simulink model "power_V__"  (R2019b)
settings: Solver=ode23tb  StartTime=0.0  StopTime=24*60*60  RelTol=1e-4  AbsTol=5e-3
PreLoadFcn:
  | % Load Data and Parameters used by the model:
  | load power_V2G.mat
  | to=0.1;
undefined symbols (not defined in the file): A, B, C, D1, Dd, Delta, j, V2G
libraries: powerlib x37, powerlib_meascontrol x5, simulink x5, spsDieselMotorModel x1, sps_avr x1, V2Glib x1, simulink_extras x1
(part 1 of 2)
settings Model: SimulationMode=accelerator  ExtModeTrigDuration=100  Creator=MathWorks  LastModifiedBy=mdeat
settings SolverCC: AutoScaleAbsTol=off  MaxConsecutiveMinStep=1e6
settings DataIOCC: LimitDataPoints=on  SaveFormat=Array  ReturnWorkspaceOutputs=off
settings OptimizationCC: BlockReduction=off  BooleanDataType=off  EfficientMapNaN2IntZero=off  LifeSpan=inf
settings DebuggingCC: SaveWithParameterizedLinksMsg=none  UnderspecifiedInitializationDetection=Classic  MergeDetectMultiDrivingBlocksExec=none  SignalResolutionControl=TryResolveAllWithWarning  AllowSymbolicDim=off  SFUnexpectedBacktrackingDiag=warning  SFNoUnconditionalDefaultTransitionDiag=warning  SFExecutionAtInitializationDiag=none  ArithmeticOperatorsInVariantConditions=warning
settings HardwareCC: ProdBitPerPointer=32  ProdBitPerSizeT=32  ProdBitPerPtrDiffT=32  ProdLargestAtomicFloat=None  ProdIntDivRoundTo=Undefined  ProdEndianess=Unspecified  ProdWordSize=32  ProdHWDeviceType=32-bit Generic  TargetBitPerPointer=64  TargetBitPerSizeT=64  TargetBitPerPtrDiffT=64  TargetLongLongMode=on  TargetIntDivRoundTo=Zero  TargetEndianess=LittleEndian  TargetWordSize=64  TargetHWDeviceType=MATLAB Host  ProdEqTarget=off
settings ModelReferenceCC: PropagateSignalLabelsOutOfModel=off
settings SFSimCC: SimUseLocalCustomCode=off  CustomCodeUndefinedFunction=UseInterfaceOnly
settings RTWCC: RTWUseLocalCustomCode=off
settings CodeAppCC: MaxIdLength=128
settings GRTTargetCC: TargetLangStandard=C89/C90 (ANSI)  CombineOutputUpdateFcns=off  GRTInterface=on
settings ConfigComp: CovMetricSettings=dw  CovHtmlReporting=on  CovSaveCumulativeToWorkspaceVar=on  CovSaveSingleToWorkspaceVar=on  CovExternalEMLEnable=off  CovSFcnEnable=off
settings SimscapeCC: SimscapeNormalizeSystem=off

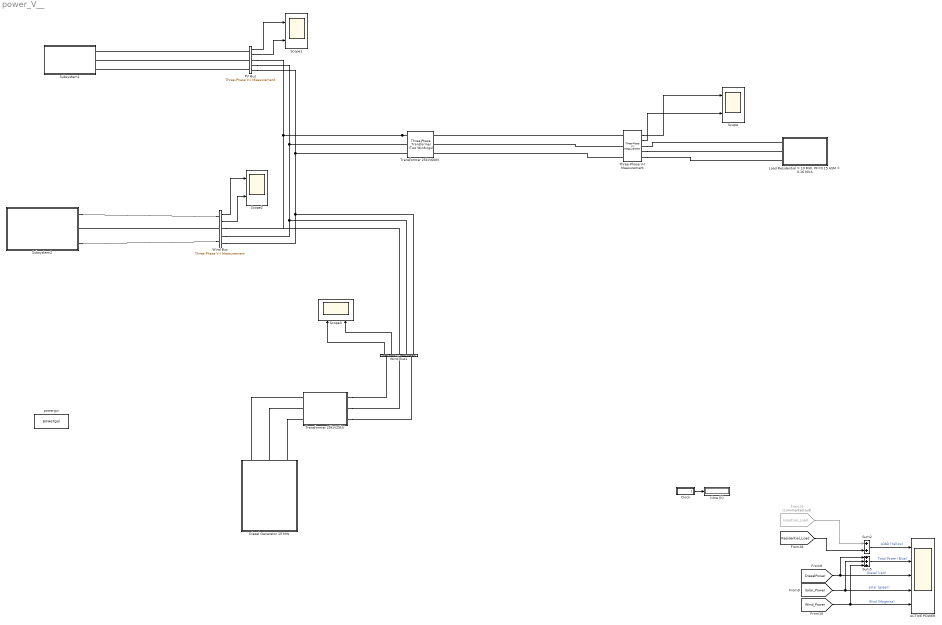
== system power_V__ ==
  ACTIVE POWER : Scope  NumInputPorts=5
  Clock : Subsystem
  Diesel Generator 15 MW : Subsystem
      mask Display: image(imread('diesel.jpg'))
  From29 : From  Commented=on  GotoTag=Industrial_Load  TagVisibility=global
  "Load Residential = 10 MW, PF=0.15 ASM = 0.16 MVA " : Subsystem
      mask Display: image(imread('load.jpg'))
  PV Bus : powerlib/Measurements/Three-Phase V-I Measurement  VoltageMeasurement=phase-to-ground  SetLabelV=off  LabelV=Vabc  Vpu=off  VpuLL=off  CurrentMeasurement=yes  SetLabelI=off  LabelI=Iabc  Ipu=off  Pbase=100e6  Vbase=500e3  OutputType=Complex  PhasorSimulation=on  PSBequivalent=0
      settings: SourceProductName=Simscape Electrical
  Scope{,1..3} (4 alike) : Scope  NumInputPorts=2
  Subsystem1 : Subsystem
  Subsystem2 : Subsystem
  Sum2 : Sum
  Sum5 : Sum  Inputs=+++
  Three-Phase V-I Measurement : powerlib/Measurements/Three-Phase V-I Measurement  VoltageMeasurement=phase-to-ground  SetLabelV=off  LabelV=Vabc  Vpu=off  VpuLL=off  CurrentMeasurement=yes  SetLabelI=off  LabelI=Iabc  Ipu=off  Pbase=100e6  Vbase=500e3  OutputType=Complex  PhasorSimulation=on  PSBequivalent=0
      settings: SourceProductName=Simscape Electrical
  Transformer 25kV/25kV : Subsystem
  Transformer 25kV/600V : powerlib/Elements/Three-Phase Transformer (Two Windings)  Winding1Connection=Yg  Winding2Connection=Yg  CoreType=Three single-phase transformers  SetSaturation=off  Hysteresis=off  DataFile='hysteresis'  SetInitialFlux=off  Measurements=None  UNITS=pu  NominalPower=[ 20e6 , 60 ]  Winding1=[25e3 ,0.002 , 0.08 ]  Winding2=[ 600 , 0.002 , 0.08 ]  Rm=500  Lm=500  L0=0.5  Saturation=[ 0,0 ; 0.0024,1.2 ; 1.0,1.52 ]  InitialFluxes=[ 0.8 , -0.8 , 0.7 ]  BreakLoop=off  DiscreteSolver=Trapezoidal iterative  DataType=off  TransfoNumber=1
      settings: SourceProductName=Simscape Electrical
  Wind Bus : powerlib/Measurements/Three-Phase V-I Measurement  VoltageMeasurement=phase-to-ground  SetLabelV=off  LabelV=Vabc  Vpu=off  VpuLL=off  CurrentMeasurement=yes  SetLabelI=off  LabelI=Iabc  Ipu=off  Pbase=100e6  Vbase=500e3  OutputType=Complex  PhasorSimulation=on  PSBequivalent=0
      settings: SourceProductName=Simscape Electrical
  Wind Bus1 : powerlib/Measurements/Three-Phase V-I Measurement  VoltageMeasurement=phase-to-ground  SetLabelV=off  LabelV=Vabc  Vpu=off  VpuLL=off  CurrentMeasurement=yes  SetLabelI=off  LabelI=Iabc  Ipu=off  Pbase=100e6  Vbase=500e3  OutputType=Complex  PhasorSimulation=on  PSBequivalent=0
      settings: SourceProductName=Simscape Electrical
  powergui : powerlib/powergui  Priority=1  SimulationMode=Phasor  SampleTime=50e-6  frequency=60  Iterations=50  frequencyindice=60  Pbase=10e6  ErrMax=0.0001  UnitsV=kV  UnitsW=MW  buscounter=0  FunctionMessages=off  echomessages=off  EnableUseOfTLC=off  CurrentSourceSwitches=off  DisableSnubberDevices=off  DisableRonSwitches=off  DisableVfSwitches=off  DisplayEquations=off  AutomaticDiscreteSolvers=off  SolverType=Tustin  Interpol=off  ExternalGateDelay=off  methode=off  Ts=100  x0status=blocks  SPID=off  SwTol=0  HookPort=off  NonlinearTolerance=0  nMaxIteration=15  ContinueOnMaxIteration=off  RestoreLinks=warning  ResistiveCurrentMeasurement=off  Frange=[0:2:500]  Ylog=off  Xlog=on  ShowGrid=off  save=off  variable=ZData  structure=0  ZoomFFT=off  StartTime=0.0  cycles=1  DisplayStyle=1  fundamental=60  FreqAxis=off  MaxFrequency=1000  frequencyindicesteady=1  RmsSteady=1  display=off
      settings: SourceProductName=Simscape Electrical
  time (h) : Display
      settings: Format=bank
  wires:
  Clock/1(" ") -> time (h)/1
  [Residential_Load] -> Sum2/2
  [Wind_Power] -> Sum5/3, ACTIVE POWER/5  "Wind (Magenta)"
  [DieselPower] -> Sum5/1, ACTIVE POWER/3  "Diesel (red)"
  [Solar_Power] -> Sum5/2, ACTIVE POWER/4  "solar (green)"
  Sum2/1 -> ACTIVE POWER/1  "LOAD (Yellow)"
  Sum5/1 -> ACTIVE POWER/2  "Total Power (Blue)"
  From29/1 -> Sum2/1
  Three-Phase V-I Measurement/1 -> Scope/1
  Three-Phase V-I Measurement/2 -> Scope/2
  PV Bus/1 -> Scope1/1
  PV Bus/2 -> Scope1/2
  Wind Bus/1 -> Scope2/1
  Wind Bus/2 -> Scope2/2
  Wind Bus1/2 -> Scope3/2
  Wind Bus1/1 -> Scope3/1
  connections:
  Three-Phase V-I Measurement/LConn2 -- Transformer 25kV/600V/RConn2
  Three-Phase V-I Measurement/LConn3 -- Transformer 25kV/600V/RConn3
  Three-Phase V-I Measurement/LConn1 -- Transformer 25kV/600V/RConn1
  Transformer 25kV/600V/LConn1 -- Wind Bus1/RConn1 -- Wind Bus/RConn1 -- PV Bus/RConn1
  Wind Bus/RConn2 -- Wind Bus1/RConn2 -- PV Bus/RConn2 -- Transformer 25kV/600V/LConn2
  Wind Bus/RConn3 -- Wind Bus1/RConn3 -- PV Bus/RConn3 -- Transformer 25kV/600V/LConn3
  Three-Phase V-I Measurement/RConn3 -- "Load Residential = 10 MW, PF=0.15 ASM = 0.16 MVA "/LConn3
  Three-Phase V-I Measurement/RConn2 -- "Load Residential = 10 MW, PF=0.15 ASM = 0.16 MVA "/LConn2
  Three-Phase V-I Measurement/RConn1 -- "Load Residential = 10 MW, PF=0.15 ASM = 0.16 MVA "/LConn1
  PV Bus/LConn1 -- Subsystem1/RConn1
  PV Bus/LConn2 -- Subsystem1/RConn2
  PV Bus/LConn3 -- Subsystem1/RConn3
  Subsystem2/RConn1 -- Wind Bus/LConn1
  Wind Bus/LConn2 -- Subsystem2/RConn2
  Subsystem2/RConn3 -- Wind Bus/LConn3
  Transformer 25kV/25kV/RConn1 -- Wind Bus1/LConn1
  Transformer 25kV/25kV/RConn2 -- Wind Bus1/LConn2
  Transformer 25kV/25kV/RConn3 -- Wind Bus1/LConn3
  Diesel Generator 15 MW/RConn1 -- Transformer 25kV/25kV/LConn1
  Diesel Generator 15 MW/RConn2 -- Transformer 25kV/25kV/LConn2
  Diesel Generator 15 MW/RConn3 -- Transformer 25kV/25kV/LConn3

== system power_V__/Clock ==
  Clock : Clock
  Gain : Gain  Gain=1/(60*60)
  " " : Outport  VectorParamsAs1DForOutWhenUnconnected=off
  wires:
  Gain/1 -> " "/1
  Clock/1 -> Gain/1

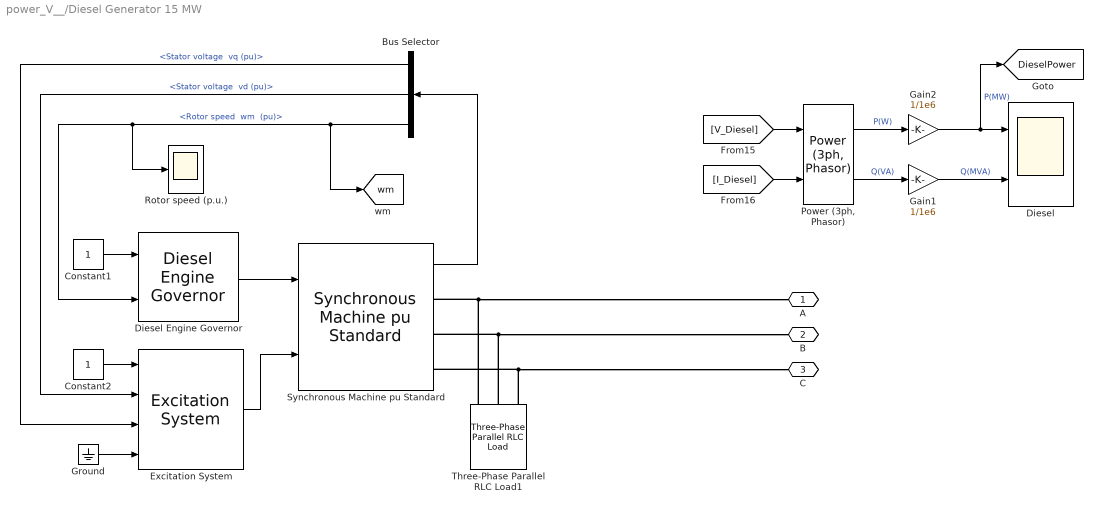
== system power_V__/Diesel Generator 15 MW ==
  Bus Selector : BusSelector  OutputSignals="dq0 components.Stator voltage  vq (pu),dq0 components.Stator voltage  vd (pu),Mechanical.Rotor speed  wm  (pu)"
  Constant1 : Constant
  Constant2 : Constant
  Diesel : Scope  NumInputPorts=2
  Diesel Engine Governor : spsDieselMotorModel/Diesel Engine Governor  K=29  Tr=[0.01 0.02 0.2]  Ta=[0.25 0.009 0.0384]  Tlim=[0 1.1]  Td=0.024  Pm0=0.007343
      settings: SourceProductName=Simscape Electrical  SourceProductBaseCode=PS
  Excitation System : sps_avr/Excitation System  tr=20e-3  reg=[ 300, 0.001 ]  exc=[ 1, 0 ]  tgr=[ 0, 0 ]  damp=[ 0.001, 0.1 ]  sat=[ 0, 0 ]  lim=[ -11.5, 11.5, 0 ]  v0=[1 1.0072]
      settings: SourceProductName=Simscape Electrical  SourceProductBaseCode=PS
  Gain1 : Gain  Gain=1/1e6
  Gain2 : Gain  Gain=1/1e6
  Ground : Ground
  "Power (3ph, Phasor)" : powerlib_meascontrol/Measurements/Power (3ph, Phasor)
      settings: SourceProductName=Simscape Electrical  SourceProductBaseCode=PS
  Rotor speed (p.u.) : Scope
  Synchronous Machine pu Standard : powerlib/Machines/Synchronous Machine pu Standard  PresetModel=No  MechanicalLoad=Mechanical power Pm  ShowDetailedParameters=on  RotorType=Salient-pole  Units=per unit standard parameters  MeasurementBus=off  NominalParameters="[ 15E6  25e3   60]"  Reactances1=[ 1.81, 0.3, 0.23, 1.76, 0.65, 0.25, 0.15 ]  Reactances2="[ 1.305, 0.296, 0.252, 0.474,  0.243,  0.18 ]"  dAxisTimeConstants=Open-circuit  qAxisTimeConstants=Short-circuit  TimeConstants1="[ 4.4849  0.0681  0.1  ]"  TimeConstants2=[ 8.0, 0.03, 1.0, 0.07 ]  TimeConstants3="[  4.49  0.0681  0.0513  ]"  TimeConstants4=[ 8.0, 0.03, 0.3371, 0.0295 ]  TimeConstants5=[ 1.01, 0.053, 0.1 ]  TimeConstants6=[ 1.3201, 0.023, 1.0, 0.07 ]  TimeConstants7=[0.012 0.003 0.003]  TimeConstants8=[ 1.3201, 0.0231, 0.3371, 0.0295 ]  StatorResistance=0.003  Mechanical=[3.7 0 1 ]  PolePairs=20  InitialConditions=[0 -89.802 0.00913935 0.00913935 0.00913935 -36.542 -156.542 83.458 1.00715]  SetSaturation=off  Saturation=[0.6404,0.7127,0.8441,0.9214,0.9956,1.082,1.19,1.316,1.457;0.7,0.7698,0.8872,0.9466,0.9969,1.046,1.1,1.151,1.201]  LoadFlowParameters=[1,0,0,0,0]  TsPowergui=0  TsBlock=-1  IterativeModel=Trapezoidal non iterative  IterativeDiscreteModel=Trapezoidal non iterative  BusType=swing  Pref=0  Qref=0  Qmin=-inf  Qmax=inf  PLF=0  QLF=0
      settings: SourceProductName=Simscape Electrical
  Three-Phase Parallel RLC Load1 : powerlib/Elements/Three-Phase Parallel RLC Load  LConnTagsString=A|B|C  Configuration=Y (floating)  NominalVoltage=(25000*sqrt(3))*1  Vabc=[1e3 1e3 1e3]  Vabcp=[1e3 1e3 1e3]  NominalFrequency=60  UnbalancedPower=off  ActivePower=1e3  InductivePower=0  CapacitivePower=0  Pabc=[10e3 9e3 11e3]  QLabc=[100 90 110]  QCabc=[100 90 110]  Pabcp=[10e3 9e3 11e3]  QLabcp=[100 90 110]  QCabcp=[100 90 110]  Measurements=None  LoadType=constant PQ
      settings: SourceProductName=Simscape Electrical
  A : PMIOPort  Side=Right
  B : PMIOPort  Port=2  Side=Right
  C : PMIOPort  Port=3  Side=Right
  tag scope: DieselPower=global, wm=global
  wires:
  Bus Selector/3 -> [wm], Rotor speed (p.u.)/1, Diesel Engine Governor/2  "<Rotor speed  wm  (pu)>"
  Constant1/1 -> Diesel Engine Governor/1
  Diesel Engine Governor/1 -> Synchronous Machine pu Standard/1
  Excitation System/1 -> Synchronous Machine pu Standard/2
  Constant2/1 -> Excitation System/1
  Bus Selector/2 -> Excitation System/2  "<Stator voltage  vd (pu)>"
  Bus Selector/1 -> Excitation System/3  "<Stator voltage  vq (pu)>"
  Synchronous Machine pu Standard/1 -> Bus Selector/1
  Ground/1 -> Excitation System/4
  Gain2/1 -> [DieselPower], Diesel/1  "P(MW)"
  "Power (3ph, Phasor)"/1 -> Gain2/1  "P(W)"
  [V_Diesel] -> "Power (3ph, Phasor)"/1
  [I_Diesel] -> "Power (3ph, Phasor)"/2
  "Power (3ph, Phasor)"/2 -> Gain1/1  "Q(VA)"
  Gain1/1 -> Diesel/2  "Q(MVA)"
  connections:
  Three-Phase Parallel RLC Load1/LConn3 -- C/RConn1 -- Synchronous Machine pu Standard/RConn3
  Three-Phase Parallel RLC Load1/LConn2 -- B/RConn1 -- Synchronous Machine pu Standard/RConn2
  Three-Phase Parallel RLC Load1/LConn1 -- A/RConn1 -- Synchronous Machine pu Standard/RConn1

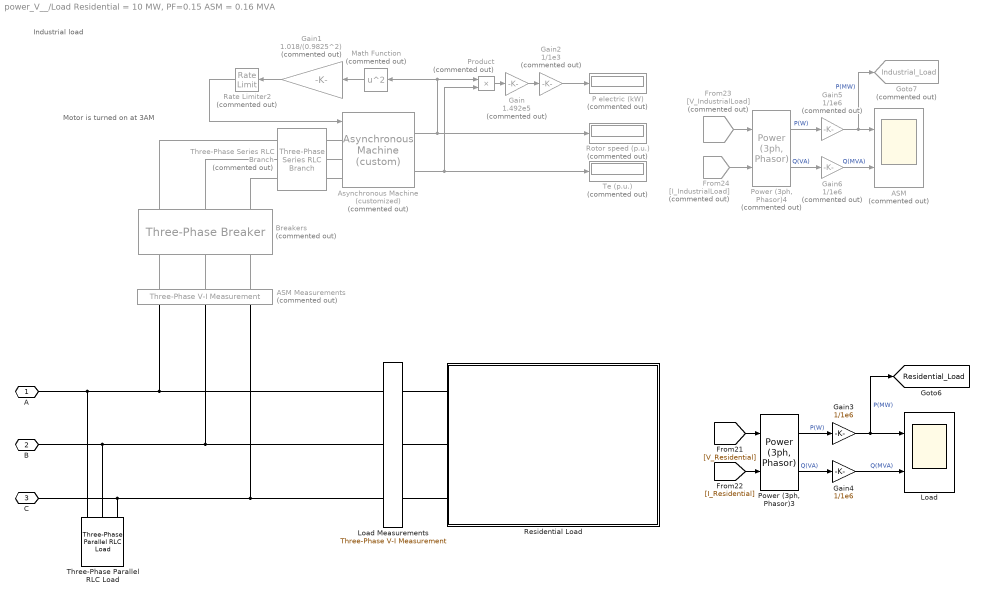
== system power_V__/Load Residential = 10 MW, PF=0.15 ASM = 0.16 MVA  ==
  note: Motor is turned on at 3AM
  note: Industrial load
  " ASM Measurements" : powerlib/Measurements/Three-Phase V-I Measurement  Commented=on  VoltageMeasurement=phase-to-ground  SetLabelV=on  LabelV=V_IndustrialLoad  Vpu=off  VpuLL=off  CurrentMeasurement=yes  SetLabelI=on  LabelI=I_IndustrialLoad  Ipu=off  Pbase=2*1.5e6/0.9  Vbase=25e3  OutputType=Complex  PhasorSimulation=on  PSBequivalent=0
      settings: SourceProductName=Simscape Electrical
  " Load Measurements" : powerlib/Measurements/Three-Phase V-I Measurement  VoltageMeasurement=phase-to-ground  SetLabelV=on  LabelV=V_Residential  Vpu=off  VpuLL=off  CurrentMeasurement=yes  SetLabelI=on  LabelI=I_Residential  Ipu=off  Pbase=2*1.5e6/0.9  Vbase=25e3  OutputType=Complex  PhasorSimulation=on  PSBequivalent=0
      settings: SourceProductName=Simscape Electrical
  ASM : Scope  Commented=on  NumInputPorts=2
  Asynchronous Machine (customized) : V2Glib/Asynchronous Machine (custom)  Commented=on  RotorType=Squirrel-cage  PresetModel=No  MechanicalLoad=Torque Tm  ShowDetailedParameters=on  ReferenceFrame=Rotor  Units=pu  MeasurementBus=on  NominalParameters=[1.5e+05 600 60]  Stator=[0.01117 0.04832]  Rotor=[0.006 0.04832]  Cage1=[0.01909 0.0397]  Cage2=[0.01909 0.0397]  Lm=2.424  Mechanical=[0.3096 0.01511 2]  PolePairs=2  InitialConditions=[1 0 0 0 0 0 -120 120]  SimulateSaturation=off  Saturation="[0.212,0.4201,0.8125,1.0979,1.4799,2.2457,3.2586,4.5763,6.4763 ;   0.5,0.7,0.9,1,1.1,1.2 ,1.3,1.4,1.5]"  LoadFlowParameters=0  TsPowergui=0  TsBlock=-1  IterativeModel=Trapezoidal non iterative  IterativeDiscreteModel=Trapezoidal non iterative  Pmec=2e6
      settings: SourceProductName=Simscape Electrical  SourceProductBaseCode=PS
  Breakers : powerlib/Elements/Three-Phase Breaker  Commented=on  InitialState=open  SwitchA=on  SwitchB=on  SwitchC=on  SwitchTimes=[ 3*3600] %Motor is turned on at 3AM  External=off  BreakerResistance=0.001  SnubberResistance=1e6  SnubberCapacitance=inf  Measurements=None
      settings: SourceProductName=Simscape Electrical
  From23 : From  Commented=on  GotoTag=V_IndustrialLoad  TagVisibility=global
  From24 : From  Commented=on  GotoTag=I_IndustrialLoad  TagVisibility=global
  Gain : Gain  Commented=on  Gain=1.492e5
  Gain1 : Gain  Commented=on  Gain=1.018/(0.9825^2)
  Gain2 : Gain  Commented=on  Gain=1/1e3
  Gain3 : Gain  Gain=1/1e6
  Gain4 : Gain  Gain=1/1e6
  Gain5 : Gain  Commented=on  Gain=1/1e6
  Gain6 : Gain  Commented=on  Gain=1/1e6
  Goto7 : Goto  Commented=on  GotoTag=Industrial_Load  TagVisibility=global
  Load : Scope  NumInputPorts=2
  Math Function : Math  Commented=on  Operator=square  SaturateOnIntegerOverflow=on
  P electric (kW) : Display  Commented=on
      settings: Format=bank
  "Power (3ph, Phasor)3" : powerlib_meascontrol/Measurements/Power (3ph, Phasor)
      settings: SourceProductName=Simscape Electrical  SourceProductBaseCode=PS
  "Power (3ph, Phasor)4" : powerlib_meascontrol/Measurements/Power (3ph, Phasor)  Commented=on
      settings: SourceProductName=Simscape Electrical  SourceProductBaseCode=PS
  Product : Product  Commented=on
  Rate Limiter2 : RateLimiter  Commented=on  RisingSlewLimit=1e4  FallingSlewLimit=-1e4  SampleTimeMode=inherited
  Residential Load : Subsystem  mask{nomPower=10, PF=0.95, timestep=60, datas=V2G.CONSUMPTION}
      mask prompts: nomPower "Nominal Power (MW)"; PF "Power factor"; timestep "Timestep (minutes)"; datas "Consumption datas"
      mask DialogControl DescGroupVar Prompt: Load profile
      mask DialogControl DescTextVar Prompt: The load profile allows you to fix a nominal power and and a power factor. It is also needed to specify the timestep used for the consumption datas. Finally, a vector expresses the consumption profile. It has to be expressed in per unit. It is imperative that the length of the vector fits with the timestep used.
      mask Display: image(imread('Residential.jpg'))
  Rotor speed (p.u.) : Display  Commented=on
      settings: Format=bank
  Te (p.u.) : Display  Commented=on
      settings: Format=bank
  Three-Phase Parallel RLC Load : powerlib/Elements/Three-Phase Parallel RLC Load  LConnTagsString=A|B|C  Configuration=Y (grounded)  NominalVoltage=(599.595)*1  Vabc=[1e3 1e3 1e3]  Vabcp=[1e3 1e3 1e3]  NominalFrequency=60  UnbalancedPower=off  ActivePower=1e3  InductivePower=0  CapacitivePower=0  Pabc=[10e3 9e3 11e3]  QLabc=[100 90 110]  QCabc=[100 90 110]  Pabcp=[10e3 9e3 11e3]  QLabcp=[100 90 110]  QCabcp=[100 90 110]  Measurements=None  LoadType=constant PQ
      settings: SourceProductName=Simscape Electrical
  Three-Phase Series RLC Branch : powerlib/Elements/Three-Phase Series RLC Branch  Commented=on  LConnTagsString=A|B|C  RConnTagsString=A|B|C  BranchType=R  Resistance=1  Inductance=1e-3  Capacitance=1e-6  Measurements=None
      settings: SourceProductName=Simscape Electrical
  A : PMIOPort  Side=Left
  B : PMIOPort  Port=2  Side=Left
  C : PMIOPort  Port=3  Side=Left
  tag scope: Residential_Load=global
  wires:
  Gain1/1 -> Rate Limiter2/1
  Asynchronous Machine (customized)/1 -> Math Function/1, Product/1, Rotor speed (p.u.)/1
  Asynchronous Machine (customized)/2 -> Product/2, Te (p.u.)/1
  Product/1 -> Gain/1
  Gain/1 -> Gain2/1
  Rate Limiter2/1 -> Asynchronous Machine (customized)/1
  Math Function/1 -> Gain1/1
  Gain2/1 -> P electric (kW)/1
  "Power (3ph, Phasor)3"/2 -> Gain4/1  "Q(VA)"
  [I_Residential] -> "Power (3ph, Phasor)3"/2
  "Power (3ph, Phasor)3"/1 -> Gain3/1  "P(W)"
  Gain3/1 -> Load/1, [Residential_Load]  "P(MW)"
  [V_Residential] -> "Power (3ph, Phasor)3"/1
  Gain4/1 -> Load/2  "Q(MVA)"
  Gain5/1 -> Goto7/1, ASM/1  "P(MW)"
  "Power (3ph, Phasor)4"/1 -> Gain5/1  "P(W)"
  From24/1 -> "Power (3ph, Phasor)4"/2
  "Power (3ph, Phasor)4"/2 -> Gain6/1  "Q(VA)"
  From23/1 -> "Power (3ph, Phasor)4"/1
  Gain6/1 -> ASM/2  "Q(MVA)"
  connections:
  Residential Load/LConn3 -- " Load Measurements"/RConn3
  Residential Load/LConn2 -- " Load Measurements"/RConn2
  Residential Load/LConn1 -- " Load Measurements"/RConn1
  Three-Phase Series RLC Branch/LConn2 -- Breakers/LConn2
  Three-Phase Series RLC Branch/LConn3 -- Breakers/LConn3
  Three-Phase Series RLC Branch/LConn1 -- Breakers/LConn1
  A/RConn1 -- Three-Phase Parallel RLC Load/LConn1 -- " ASM Measurements"/LConn1 -- " Load Measurements"/LConn1
  B/RConn1 -- Three-Phase Parallel RLC Load/LConn2 -- " ASM Measurements"/LConn2 -- " Load Measurements"/LConn2
  C/RConn1 -- Three-Phase Parallel RLC Load/LConn3 -- " ASM Measurements"/LConn3 -- " Load Measurements"/LConn3
  " ASM Measurements"/RConn3 -- Breakers/RConn3
  " ASM Measurements"/RConn2 -- Breakers/RConn2
  " ASM Measurements"/RConn1 -- Breakers/RConn1
  Three-Phase Series RLC Branch/RConn1 -- Asynchronous Machine (customized)/LConn1
  Three-Phase Series RLC Branch/RConn2 -- Asynchronous Machine (customized)/LConn2
  Three-Phase Series RLC Branch/RConn3 -- Asynchronous Machine (customized)/LConn3

== system power_V__/Subsystem1 ==
  PV Farm 8 MW : Subsystem  mask{eff=10, area=8e4}
      mask prompts: eff "Efficiency (%)"; area "Area (m^2)"
      mask help: The product of the effeciency, the area covered by the Pv farm and the irradiance in w/m2 will give you the power generate by the PV farm.
      mask DialogControl DescGroupVar Prompt: PV farm
      mask DialogControl DescTextVar Prompt: The product of the efficiency, the area covered by the PV farm and the irradiance in W/m2 will give you the power generated by the PV farm.
      mask Display: image(imread('panel.jpg'))
  Subsystem : Subsystem
  Conn1 : PMIOPort  Side=Right
  Conn2 : PMIOPort  Port=2  Side=Right
  Conn3 : PMIOPort  Port=3  Side=Right
  wires:
  Subsystem/1(Out1) -> PV Farm 8 MW/1(Irradiance)
  connections:
  Conn1/RConn1 -- PV Farm 8 MW/RConn1
  Conn2/RConn1 -- PV Farm 8 MW/RConn2
  Conn3/RConn1 -- PV Farm 8 MW/RConn3

== system power_V__/Subsystem2 ==
  Subsystem : Subsystem
  Wind Farm 4.5 MW : Subsystem  mask{nomPower=4.5, nomwind=13.5, maxwind=15}
      mask prompts: nomPower "Nominal power (MW)"; nomwind "Nominal wind speed (m/s)"; maxwind "Maximal wind speed (m/s)"
      mask DialogControl DescGroupVar Prompt: Wind farm
      mask DialogControl DescTextVar Prompt: The simplified wind farm model presented here generates power using a linear relationship between the nominal wind speed and nominal power. When the wind speed reaches the maximal value, the wind farm trips from the grid. When the wind speed is between the nominal speed and the maximal value, the power is fixed to 1 p.u.
      mask Display: image(imread('windfarm.jpg'))
  Conn1 : PMIOPort  Side=Right
  Conn2 : PMIOPort  Port=2  Side=Right
  Conn3 : PMIOPort  Port=3  Side=Right
  wires:
  Subsystem/1(Out1) -> Wind Farm 4.5 MW/1(wind)
  connections:
  Wind Farm 4.5 MW/RConn1 -- Conn1/RConn1
  Conn2/RConn1 -- Wind Farm 4.5 MW/RConn2
  Wind Farm 4.5 MW/RConn3 -- Conn3/RConn1

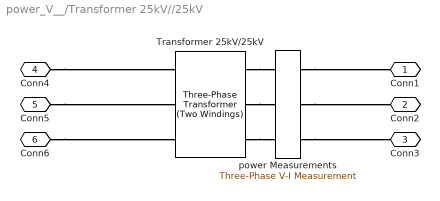
== system power_V__/Transformer 25kV//25kV ==
  " power Measurements" : powerlib/Measurements/Three-Phase V-I Measurement  VoltageMeasurement=phase-to-ground  SetLabelV=on  LabelV=V_Diesel  Vpu=off  VpuLL=off  CurrentMeasurement=yes  SetLabelI=on  LabelI=I_Diesel  Ipu=off  Pbase=2*1.5e6/0.9  Vbase=25e3  OutputType=Complex  PhasorSimulation=on  PSBequivalent=0
      settings: SourceProductName=Simscape Electrical
  Transformer 25kV/25kV : powerlib/Elements/Three-Phase Transformer (Two Windings)  Winding1Connection=Delta (D1)  Winding2Connection=Yg  CoreType=Three single-phase transformers  SetSaturation=off  Hysteresis=off  DataFile='hysteresis'  SetInitialFlux=off  Measurements=None  UNITS=pu  NominalPower=[ 20e6 , 60 ]  Winding1=[25e3 , 0.002 , 0.08 ]  Winding2=[ 25e3 , 0.002 , 0.08 ]  Rm=500  Lm=500  L0=0.5  Saturation=[ 0,0 ; 0.0024,1.2 ; 1.0,1.52 ]  InitialFluxes=[ 0.8 , -0.8 , 0.7 ]  BreakLoop=off  DiscreteSolver=Trapezoidal iterative  DataType=off  TransfoNumber=1
      settings: SourceProductName=Simscape Electrical
  Conn1 : PMIOPort  Side=Right
  Conn2 : PMIOPort  Port=2  Side=Right
  Conn3 : PMIOPort  Port=3  Side=Right
  Conn4 : PMIOPort  Port=4  Side=Left
  Conn5 : PMIOPort  Port=5  Side=Left
  Conn6 : PMIOPort  Port=6  Side=Left
  connections:
  " power Measurements"/RConn3 -- Conn3/RConn1
  " power Measurements"/RConn2 -- Conn2/RConn1
  Conn4/RConn1 -- Transformer 25kV/25kV/LConn1
  Transformer 25kV/25kV/RConn3 -- " power Measurements"/LConn3
  Transformer 25kV/25kV/RConn2 -- " power Measurements"/LConn2
  Conn6/RConn1 -- Transformer 25kV/25kV/LConn3
  Conn5/RConn1 -- Transformer 25kV/25kV/LConn2
  Transformer 25kV/25kV/RConn1 -- " power Measurements"/LConn1
  " power Measurements"/RConn1 -- Conn1/RConn1

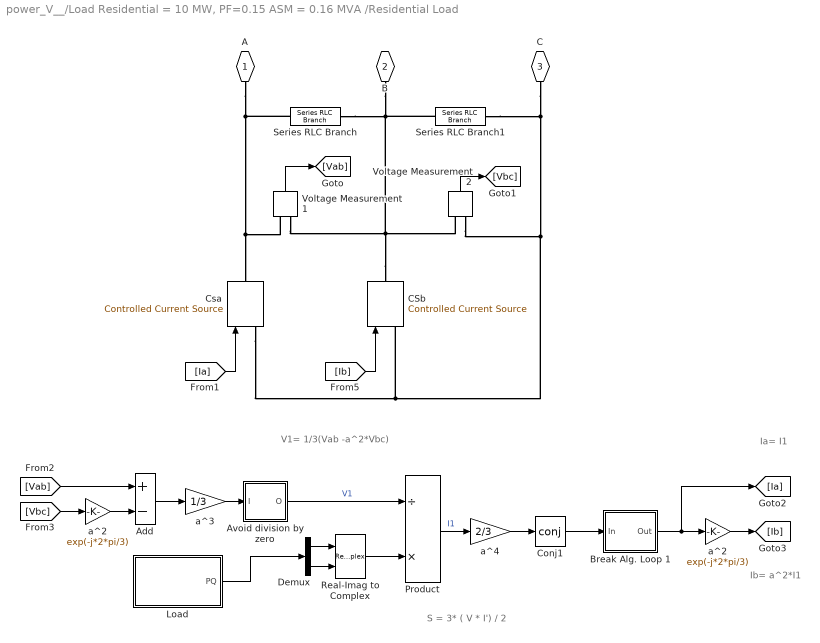
== system power_V__/Load Residential = 10 MW, PF=0.15 ASM = 0.16 MVA /Residential Load ==
  note: V1= 1/3(Vab -a^2*Vbc)
  note: S = 3* ( V * I') / 2
  note: Ia= I1
  note: Ib= a^2*I1
  Add : Sum  Inputs=+-
  Avoid division by zero : Subsystem
  Break Alg. Loop 1 : Subsystem
  CSb : powerlib/Electrical Sources/Controlled Current Source  Initialize=on  Source_Type=AC  Amplitude=9355.5  Phase=(2.751-2*pi/3)*180/pi  Frequency=60  Measurements=Current
      settings: SourceProductName=Simscape Electrical
  Conj1 : Math  Operator=conj  SaturateOnIntegerOverflow=on
  Csa : powerlib/Electrical Sources/Controlled Current Source  Initialize=on  Source_Type=AC  Amplitude=9355.5  Phase=2.751*180/pi  Frequency=60  Measurements=Current
      settings: SourceProductName=Simscape Electrical
  Demux : Demux  Outputs=2
  Load : Subsystem
  Product : Product  Inputs=/*  SaturateOnIntegerOverflow=on  InputSameDT=on  OutDataTypeStr=Inherit: Same as first input
  Real-Imag to Complex : RealImagToComplex
  Series RLC Branch : powerlib/Elements/Series RLC Branch  LConnTagsString=__new0  RConnTagsString=__new0  BranchType=R  Resistance=1e6  Inductance=1e-3  SetiL0=off  InitialCurrent=0  Capacitance=1e-6  Setx0=off  InitialVoltage=0  Measurements=None
      settings: SourceProductName=Simscape Electrical
  Series RLC Branch1 : powerlib/Elements/Series RLC Branch  LConnTagsString=__new0  RConnTagsString=__new0  BranchType=R  Resistance=1e6  Inductance=1e-3  SetiL0=off  InitialCurrent=0  Capacitance=1e-6  Setx0=off  InitialVoltage=0  Measurements=None
      settings: SourceProductName=Simscape Electrical
  Voltage Measurement1 : powerlib/Measurements/Voltage Measurement  PhasorSimulation=on  OutputType=Complex  PSBequivalent=0
      settings: SourceProductName=Simscape Electrical
  Voltage Measurement2 : powerlib/Measurements/Voltage Measurement  PhasorSimulation=on  OutputType=Complex  PSBequivalent=0
      settings: SourceProductName=Simscape Electrical
  a^2 : Gain  Gain=exp(-j*2*pi/3)  SaturateOnIntegerOverflow=on  OutDataTypeStr=Inherit: Same as input  ParamDataTypeStr=Inherit: Same as input
  "a^2 " : Gain  Gain=exp(-j*2*pi/3)  SaturateOnIntegerOverflow=on  OutDataTypeStr=Inherit: Same as input  ParamDataTypeStr=Inherit: Same as input
  a^3 : Gain  Gain=1/3  SaturateOnIntegerOverflow=on  OutDataTypeStr=Inherit: Same as input  ParamDataTypeStr=Inherit: Same as input
  a^4 : Gain  Gain=2/3  SaturateOnIntegerOverflow=on  OutDataTypeStr=Inherit: Same as input  ParamDataTypeStr=Inherit: Same as input
  A : PMIOPort  Tag=PMCPort  Side=Left
  B : PMIOPort  Tag=PMCPort  Port=2  Side=Left
  C : PMIOPort  Tag=PMCPort  Port=3  Side=Left
  wires:
  Voltage Measurement1/1 -> [Vab]
  Voltage Measurement2/1 -> [Vbc]
  [Ia] -> Csa/1
  [Ib] -> CSb/1
  Real-Imag to Complex/1 -> Product/2
  Product/1 -> a^4/1  "I1"
  a^2/1 -> [Ib]
  a^3/1 -> Avoid division by zero/1(I)
  Add/1 -> a^3/1
  [Vab] -> Add/1
  [Vbc] -> "a^2 "/1
  "a^2 "/1 -> Add/2
  a^4/1 -> Conj1/1
  Demux/1 -> Real-Imag to Complex/1
  Demux/2 -> Real-Imag to Complex/2
  Load/1(PQ) -> Demux/1
  Avoid division by zero/1(O) -> Product/1  "V1"
  Conj1/1 -> Break Alg. Loop 1/1(In)
  Break Alg. Loop 1/1(Out) -> [Ia], a^2/1
  connections:
  Series RLC Branch/LConn1 -- A/RConn1 -- Csa/RConn1 -- Voltage Measurement1/LConn1
  Voltage Measurement2/LConn2 -- C/RConn1 -- Series RLC Branch1/RConn1 -- Csa/LConn1 -- CSb/LConn1
  CSb/RConn1 -- Voltage Measurement2/LConn1 -- Voltage Measurement1/LConn2 -- B/RConn1 -- Series RLC Branch1/LConn1 -- Series RLC Branch/RConn1

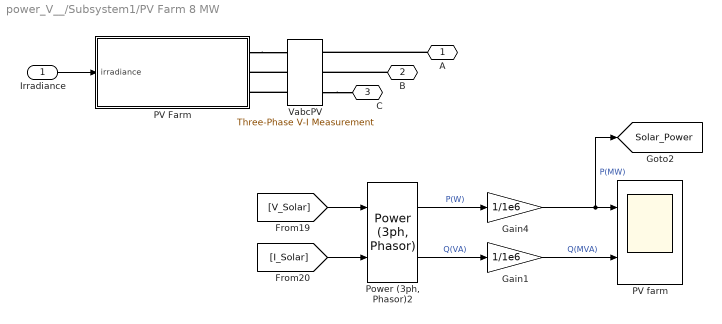
== system power_V__/Subsystem1/PV Farm 8 MW ==
  Irradiance : Inport
  Gain1 : Gain  Gain=1/1e6
  Gain4 : Gain  Gain=1/1e6
  PV Farm : Subsystem
  PV farm : Scope  NumInputPorts=2
  "Power (3ph, Phasor)2" : powerlib_meascontrol/Measurements/Power (3ph, Phasor)
      settings: SourceProductName=Simscape Electrical  SourceProductBaseCode=PS
  VabcPV : powerlib/Measurements/Three-Phase V-I Measurement  VoltageMeasurement=phase-to-ground  SetLabelV=on  LabelV=V_Solar  Vpu=off  VpuLL=off  CurrentMeasurement=yes  SetLabelI=on  LabelI=I_Solar  Ipu=off  Pbase=2*1.5e6/0.9  Vbase=25e3  OutputType=Complex  PhasorSimulation=on  PSBequivalent=0
      settings: SourceProductName=Simscape Electrical
  A : PMIOPort  Side=Right
  B : PMIOPort  Port=2  Side=Right
  C : PMIOPort  Port=3  Side=Right
  tag scope: Solar_Power=global
  wires:
  Irradiance/1 -> PV Farm/1(irradiance)
  [V_Solar] -> "Power (3ph, Phasor)2"/1
  "Power (3ph, Phasor)2"/1 -> Gain4/1  "P(W)"
  [I_Solar] -> "Power (3ph, Phasor)2"/2
  "Power (3ph, Phasor)2"/2 -> Gain1/1  "Q(VA)"
  Gain4/1 -> [Solar_Power], PV farm/1  "P(MW)"
  Gain1/1 -> PV farm/2  "Q(MVA)"
  connections:
  B/RConn1 -- VabcPV/RConn2
  VabcPV/LConn2 -- PV Farm/RConn2
  A/RConn1 -- VabcPV/RConn1
  VabcPV/RConn3 -- C/RConn1
  PV Farm/RConn1 -- VabcPV/LConn1
  VabcPV/LConn3 -- PV Farm/RConn3

== system power_V__/Subsystem1/Subsystem ==
  Irradiance : Subsystem
      mask init:
      | load power_V2G
      mask Display: plot(V2G.IRRADIANCE.time,V2G.IRRADIANCE.SUN)
  Partial Shading : Subsystem  mask(Signal Disturbance){Hour=12, Minute=0, Second=0, Duration=5*60, Factor=0.7}
      mask prompts: Duration "Duration (s):"
      mask help: Within the specified time range defined by Start and Duration parameters, output is set to 'Factor'. Outside the specified time range output is kept at 1.0.
      mask init:
      | T2=(Hour-1)*60*60;    % Hour in seconds
      | T3=(Minute-1)*60;  % Minute in seconds
      | Ton=T2+T3+(Second-1);    % Beginning of fault (s)
      | Toff=Ton+Duration; % End of fault (s)
      mask TypeOptions Hour: 0 |      1 |      2 |      3 |      4 |      5 |      6 |      7 |      8 |      9 |     10 |     11 |     12 |     13 |     14 |     15 |     16 |     17 |     18 |     19 |     20 |     21 |     22 |     23
      mask TypeOptions Minute: 0 |      1 |      2 |      3 |      4 |      5 |      6 |      7 |      8 |      9 |     10 |     11 |     12 |     13 |     14 |     15 |     16 |     17 |     18 |     19 |     20 |     21 |     22 |     23 |     24 |     25 |     26 |     27 |     28 |     29 |     30 |     31 |     32 |     33 |     34 |     35 |     36 |     37 |     38 |     39 |     40 |     41 |     42 |     43 |     44 |     45 |     46 |     47 |     48 |     49 |     50 |     51 |     52 |     53 |     54 |     55 |     56 |     57 |     58 |     59
      mask TypeOptions Second: 0 |      1 |      2 |      3 |      4 |      5 |      6 |      7 |      8 |      9 |     10 |     11 |     12 |     13 |     14 |     15 |     16 |     17 |     18 |     19 |     20 |     21 |     22 |     23 |     24 |     25 |     26 |     27 |     28 |     29 |     30 |     31 |     32 |     33 |     34 |     35 |     36 |     37 |     38 |     39 |     40 |     41 |     42 |     43 |     44 |     45 |     46 |     47 |     48 |     49 |     50 |     51 |     52 |     53 |     54 |     55 |     56 |     57 |     58 |     59
      mask DialogControl Control2 Prompt: Start:
  Product1 : Product
  Rate Limiter2 : RateLimiter  RisingSlewLimit=1e4  FallingSlewLimit=-1e4  SampleTimeMode=inherited
  Out1 : Outport
  wires:
  Product1/1 -> Rate Limiter2/1
  Partial Shading/1(Out) -> Product1/2
  Irradiance/1(" ") -> Product1/1
  Rate Limiter2/1 -> Out1/1

== system power_V__/Subsystem2/Subsystem ==
  Wind profile : Subsystem
      mask init:
      | load power_V2G
      mask Display: plot(V2G.WINDTURBINE.time,V2G.WINDTURBINE.wind)
  Out1 : Outport
  wires:
  Wind profile/1(" ") -> Out1/1

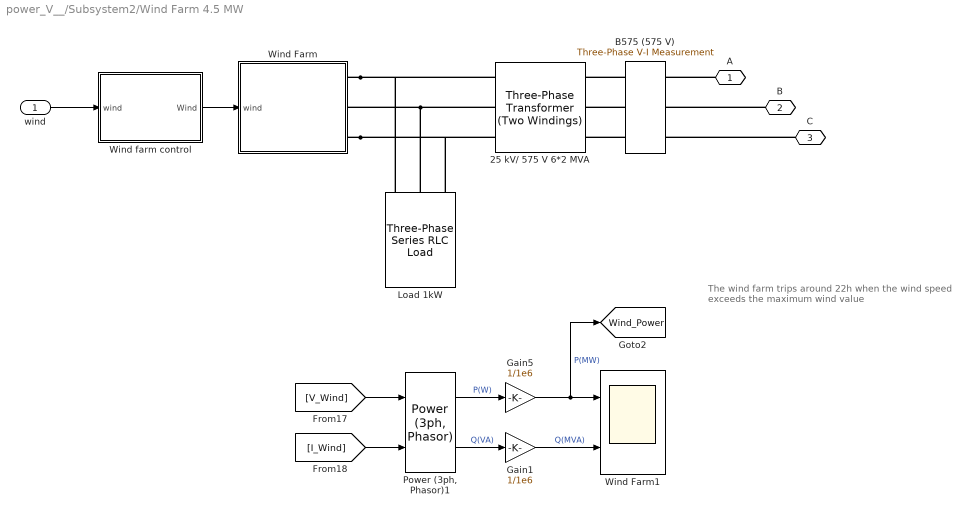
== system power_V__/Subsystem2/Wind Farm 4.5 MW ==
  note: The wind farm trips around 22h when the
      | wind speed exceeds the maximum wind value
  wind : Inport
  25 kV/ 575 V 6*2 MVA : powerlib/Elements/Three-Phase Transformer (Two Windings)  Winding1Connection=Yg  Winding2Connection=Delta (D1)  CoreType=Three single-phase transformers  SetSaturation=off  Hysteresis=off  DataFile='hysteresis'  SetInitialFlux=off  Measurements=None  UNITS=pu  NominalPower="[6*2e6  60]"  Winding1=[25e3 , 0.025/30 , 0.025]  Winding2=[ 575, 0.025/30 , 0.025]  Rm=500  Lm=inf  L0=0.5  Saturation=[ 0,0 ; 0.0024,1.2 ; 1.0,1.52 ]  InitialFluxes=[ 0.8 , -0.8 , 0.7 ]  BreakLoop=off  DiscreteSolver=Trapezoidal iterative  DataType=off  TransfoNumber=0
      settings: SourceProductName=Simscape Electrical
  B575 (575 V) : powerlib/Measurements/Three-Phase V-I Measurement  VoltageMeasurement=phase-to-ground  SetLabelV=on  LabelV=V_Wind  Vpu=off  VpuLL=off  CurrentMeasurement=yes  SetLabelI=on  LabelI=I_Wind  Ipu=off  Pbase=6*1.5e6/0.9  Vbase=575  OutputType=Complex  PhasorSimulation=on  PSBequivalent=0
      settings: SourceProductName=Simscape Electrical
  Gain1 : Gain  Gain=1/1e6
  Gain5 : Gain  Gain=1/1e6
  Load 1kW : powerlib/Elements/Three-Phase Series RLC Load  LConnTagsString=A|B|C  Configuration=Y (grounded)  NominalVoltage=(574.706)*1  Vabc=[1e3 1e3 1e3]  Vabcp=[1e3 1e3 1e3]  NominalFrequency=60  UnbalancedPower=off  ActivePower=1e3  InductivePower=0  CapacitivePower=0  Pabc=[10e3 9e3 11e3]  QLabc=[100 90 110]  QCabc=[100 90 110]  Pabcp=[10e3 9e3 11e3]  QLabcp=[100 90 110]  QCabcp=[100 90 110]  Measurements=None  LoadType=constant PQ
      settings: SourceProductName=Simscape Electrical
  "Power (3ph, Phasor)1" : powerlib_meascontrol/Measurements/Power (3ph, Phasor)
      settings: SourceProductName=Simscape Electrical  SourceProductBaseCode=PS
  Wind Farm : Subsystem
  Wind Farm1 : Scope  NumInputPorts=2
  Wind farm control : Subsystem
  A : PMIOPort  Side=Right
  B : PMIOPort  Port=2  Side=Right
  C : PMIOPort  Port=3  Side=Right
  tag scope: Wind_Power=global
  wires:
  Wind farm control/1(Wind) -> Wind Farm/1("wind ")
  wind/1 -> Wind farm control/1("wind ")
  "Power (3ph, Phasor)1"/1 -> Gain5/1  "P(W)"
  [I_Wind] -> "Power (3ph, Phasor)1"/2
  Gain5/1 -> [Wind_Power], Wind Farm1/1  "P(MW)"
  [V_Wind] -> "Power (3ph, Phasor)1"/1
  "Power (3ph, Phasor)1"/2 -> Gain1/1  "Q(VA)"
  Gain1/1 -> Wind Farm1/2  "Q(MVA)"
  connections:
  Load 1kW/LConn2 -- 25 kV/ 575 V 6*2 MVA/RConn2 -- Wind Farm/RConn2
  Wind Farm/RConn1 -- 25 kV/ 575 V 6*2 MVA/RConn1 -- Load 1kW/LConn1
  Wind Farm/RConn3 -- 25 kV/ 575 V 6*2 MVA/RConn3 -- Load 1kW/LConn3
  B575 (575 V)/LConn1 -- 25 kV/ 575 V 6*2 MVA/LConn1
  B575 (575 V)/LConn2 -- 25 kV/ 575 V 6*2 MVA/LConn2
  B575 (575 V)/LConn3 -- 25 kV/ 575 V 6*2 MVA/LConn3
  C/RConn1 -- B575 (575 V)/RConn3
  B/RConn1 -- B575 (575 V)/RConn2
  A/RConn1 -- B575 (575 V)/RConn1

== system power_V__/Load Residential = 10 MW, PF=0.15 ASM = 0.16 MVA /Residential Load/Avoid division by zero ==
  I : Inport
  Complex to Magnitude-Angle : ComplexToMagnitudeAngle
  Magnitude-Angle to Complex : MagnitudeAngleToComplex
  Saturation1 : Saturate  UpperLimit=inf  LowerLimit=1e-6
  O : Outport  VectorParamsAs1DForOutWhenUnconnected=off
  wires:
  I/1 -> Complex to Magnitude-Angle/1
  Saturation1/1 -> Magnitude-Angle to Complex/1
  Complex to Magnitude-Angle/1 -> Saturation1/1
  Magnitude-Angle to Complex/1 -> O/1
  Complex to Magnitude-Angle/2 -> Magnitude-Angle to Complex/2

== system power_V__/Load Residential = 10 MW, PF=0.15 ASM = 0.16 MVA /Residential Load/Break Alg. Loop 1 ==
  In : Inport
  Complex to Real-Imag : ComplexToRealImag
  Real-Imag to Complex : RealImagToComplex
  imag : Subsystem  mask(Transfer Function with Initial Outputs){N=[1], D=[to  1], Y0=0, U0=0}
      mask prompts: N "Numerator:"; D "Denominator:"; Y0 "Initial output:"; U0 "Initial input:"
      mask help: Vector expressions for numerator, and denominator. Coefficients are in descending powers of s.
      mask init:
      | [A,B,C,Dd]=tf2ss(N,D);if (isempty(Y0));[m,n]=size(A);X0=zeros(1,m); end; if (isempty(U0));[m,p]=size(B);U0=zeros(1,p);end;X0=getxo(A,B,C,Dd,U0,Y0,0);
      mask Help: Specify the initial output for the transfer function.  An optimization routine attempts to determine the appropriate initial states so that the specified initial output is achieved.  For more details, see the m-file getxo.m
      mask Display: dpoly(N,D,'s')
  real : Subsystem  mask(Transfer Function with Initial Outputs){N=[1], D=[to 1], Y0=0, U0=0}
      mask prompts: N "Numerator:"; D "Denominator:"; Y0 "Initial output:"; U0 "Initial input:"
      mask help: Vector expressions for numerator, and denominator. Coefficients are in descending powers of s.
      mask init:
      | [A,B,C,Dd]=tf2ss(N,D);if (isempty(Y0));[m,n]=size(A);X0=zeros(1,m); end; if (isempty(U0));[m,p]=size(B);U0=zeros(1,p);end;X0=getxo(A,B,C,Dd,U0,Y0,0);
      mask Help: Specify the initial output for the transfer function.  An optimization routine attempts to determine the appropriate initial states so that the specified initial output is achieved.  For more details, see the m-file getxo.m
      mask Display: dpoly(N,D,'s')
  Out : Outport  VectorParamsAs1DForOutWhenUnconnected=off
  wires:
  Complex to Real-Imag/1 -> real/1(In1)
  Complex to Real-Imag/2 -> imag/1(In1)
  In/1 -> Complex to Real-Imag/1
  Real-Imag to Complex/1 -> Out/1
  real/1(Out1) -> Real-Imag to Complex/1
  imag/1(Out1) -> Real-Imag to Complex/2

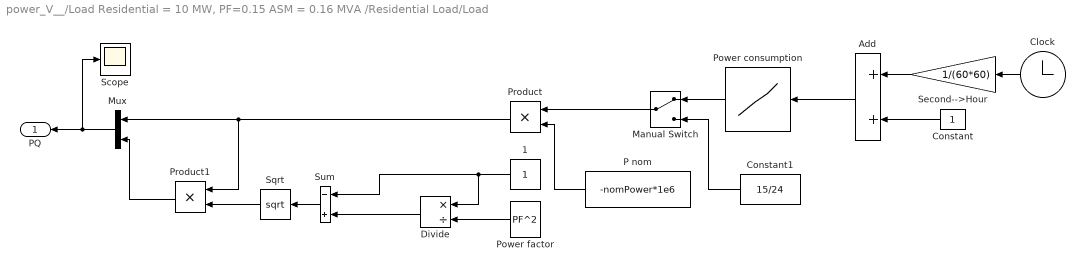
== system power_V__/Load Residential = 10 MW, PF=0.15 ASM = 0.16 MVA /Residential Load/Load ==
  1 : Constant
  Add : Sum
  Clock : Clock
  Constant : Constant
  Constant1 : Constant  Value=15/24
  Divide : Product  Inputs=*/
  Manual Switch : ManualSwitch
  Mux : Mux  Inputs=2
  P nom : Constant  Value=-nomPower*1e6
  Power consumption : Lookup_n-D  NumberOfTableDimensions=1  BreakpointsForDimension1=[1:timestep/60:24]  BeginIndexSearchUsingPreviousIndexResult=on  Table=datas  InternalRulePriority=Speed  RndMeth=Simplest  InputSameDT=on
  Power factor : Constant  Value=PF^2
  Product : Product
  Product1 : Product
  Scope : Scope
  Second-->Hour : Gain  Gain=1/(60*60)
  Sqrt : Sqrt  SaturateOnIntegerOverflow=on
  Sum : Sum  Inputs=-+
  PQ : Outport  VectorParamsAs1DForOutWhenUnconnected=off
  wires:
  Constant/1 -> Add/2
  1/1 -> Sum/1, Divide/1
  Second-->Hour/1 -> Add/1
  Sum/1 -> Sqrt/1
  Power factor/1 -> Divide/2
  Add/1 -> Power consumption/1
  P nom/1 -> Product/2
  Clock/1 -> Second-->Hour/1
  Sqrt/1 -> Product1/2
  Product/1 -> Product1/1, Mux/1
  Divide/1 -> Sum/2
  Product1/1 -> Mux/2
  Power consumption/1 -> Manual Switch/1
  Manual Switch/1 -> Product/1
  Constant1/1 -> Manual Switch/2
  Mux/1 -> Scope/1, PQ/1

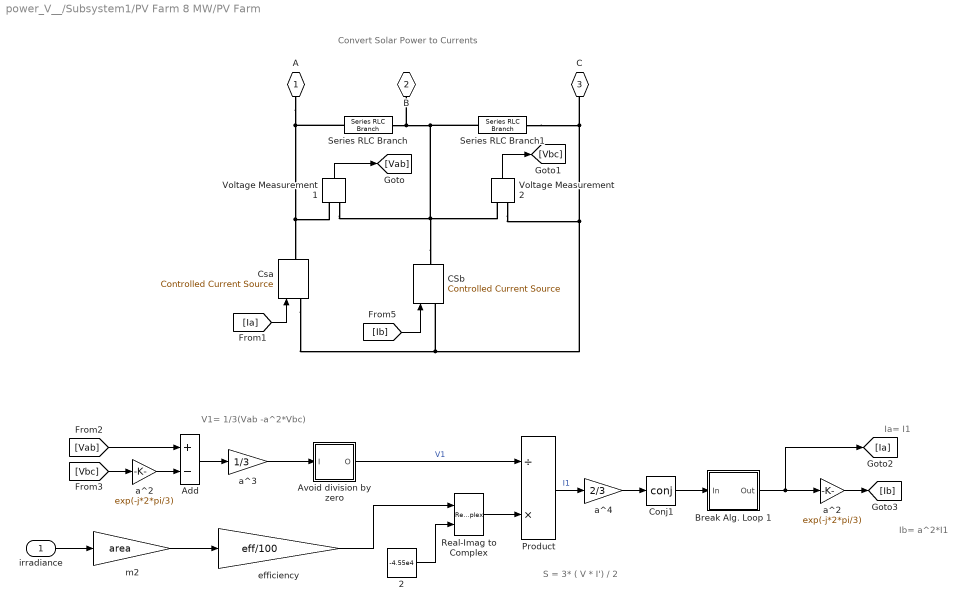
== system power_V__/Subsystem1/PV Farm 8 MW/PV Farm ==
  note: Ib= a^2*I1
  note: Ia= I1
  note: S = 3* ( V * I') / 2
  note: V1= 1/3(Vab -a^2*Vbc)
  note: Convert Solar Power to Currents
  irradiance : Inport
  2 : Constant  Value=-4.55e4
  Add : Sum  Inputs=+-
  Avoid division by zero : Subsystem
  Break Alg. Loop 1 : Subsystem
  CSb : powerlib/Electrical Sources/Controlled Current Source  Initialize=on  Source_Type=AC  Amplitude=0  Phase=0  Frequency=60  Measurements=None
      settings: SourceProductName=Simscape Electrical
  Conj1 : Math  Operator=conj  SaturateOnIntegerOverflow=on
  Csa : powerlib/Electrical Sources/Controlled Current Source  Initialize=on  Source_Type=AC  Amplitude=0  Phase=0  Frequency=60  Measurements=None
      settings: SourceProductName=Simscape Electrical
  Product : Product  Inputs=/*  SaturateOnIntegerOverflow=on  InputSameDT=on  OutDataTypeStr=Inherit: Same as first input
  Real-Imag to Complex : RealImagToComplex
  Series RLC Branch : powerlib/Elements/Series RLC Branch  LConnTagsString=__new0  RConnTagsString=__new0  BranchType=R  Resistance=1e6  Inductance=1e-3  SetiL0=off  InitialCurrent=0  Capacitance=1e-6  Setx0=off  InitialVoltage=0  Measurements=None
      settings: SourceProductName=Simscape Electrical
  Series RLC Branch1 : powerlib/Elements/Series RLC Branch  LConnTagsString=__new0  RConnTagsString=__new0  BranchType=R  Resistance=1e6  Inductance=1e-3  SetiL0=off  InitialCurrent=0  Capacitance=1e-6  Setx0=off  InitialVoltage=0  Measurements=None
      settings: SourceProductName=Simscape Electrical
  Voltage Measurement1 : powerlib/Measurements/Voltage Measurement  PhasorSimulation=on  OutputType=Complex  PSBequivalent=0
      settings: SourceProductName=Simscape Electrical
  Voltage Measurement2 : powerlib/Measurements/Voltage Measurement  PhasorSimulation=on  OutputType=Complex  PSBequivalent=0
      settings: SourceProductName=Simscape Electrical
  a^2 : Gain  Gain=exp(-j*2*pi/3)  SaturateOnIntegerOverflow=on  OutDataTypeStr=Inherit: Same as input  ParamDataTypeStr=Inherit: Same as input
  "a^2 " : Gain  Gain=exp(-j*2*pi/3)  SaturateOnIntegerOverflow=on  OutDataTypeStr=Inherit: Same as input  ParamDataTypeStr=Inherit: Same as input
  a^3 : Gain  Gain=1/3  SaturateOnIntegerOverflow=on  OutDataTypeStr=Inherit: Same as input  ParamDataTypeStr=Inherit: Same as input
  a^4 : Gain  Gain=2/3  SaturateOnIntegerOverflow=on  OutDataTypeStr=Inherit: Same as input  ParamDataTypeStr=Inherit: Same as input
  efficiency : Gain  Gain=eff/100
  m2 : Gain  Gain=area
  A : PMIOPort  Tag=PMCPort  Side=Right
  B : PMIOPort  Tag=PMCPort  Port=2  Side=Right
  C : PMIOPort  Tag=PMCPort  Port=3  Side=Right
  wires:
  [Ib] -> CSb/1
  Break Alg. Loop 1/1(Out) -> a^2/1, [Ia]
  a^4/1 -> Conj1/1
  "a^2 "/1 -> Add/2
  [Vbc] -> "a^2 "/1
  [Vab] -> Add/1
  Add/1 -> a^3/1
  a^3/1 -> Avoid division by zero/1(I)
  Conj1/1 -> Break Alg. Loop 1/1(In)
  Avoid division by zero/1(O) -> Product/1  "V1"
  a^2/1 -> [Ib]
  [Ia] -> Csa/1
  Product/1 -> a^4/1  "I1"
  Real-Imag to Complex/1 -> Product/2
  Voltage Measurement2/1 -> [Vbc]
  Voltage Measurement1/1 -> [Vab]
  efficiency/1 -> Real-Imag to Complex/1
  2/1 -> Real-Imag to Complex/2
  m2/1 -> efficiency/1
  irradiance/1 -> m2/1
  connections:
  CSb/RConn1 -- Voltage Measurement1/LConn2 -- Voltage Measurement2/LConn1 -- Series RLC Branch/RConn1 -- B/RConn1 -- Series RLC Branch1/LConn1
  Voltage Measurement2/LConn2 -- Csa/LConn1 -- CSb/LConn1 -- C/RConn1 -- Series RLC Branch1/RConn1
  A/RConn1 -- Series RLC Branch/LConn1 -- Voltage Measurement1/LConn1 -- Csa/RConn1

== system power_V__/Subsystem1/Subsystem/Irradiance ==
  1-D Lookup IRRADIANCE Table : Lookup_n-D  NumberOfTableDimensions=1  BreakpointsForDimension1=V2G.IRRADIANCE.time  BeginIndexSearchUsingPreviousIndexResult=on  Table=V2G.IRRADIANCE.SUN  InternalRulePriority=Speed  RndMeth=Simplest  InputSameDT=on
  Add : Sum
  Clock1 : Clock
  Constant1 : Constant
  Second-->Hour : Gain  Gain=1/(60*60)
  " " : Outport  VectorParamsAs1DForOutWhenUnconnected=off
  wires:
  Constant1/1 -> Add/2
  Add/1 -> 1-D Lookup IRRADIANCE Table/1  "Hour of the day"
  1-D Lookup IRRADIANCE Table/1 -> " "/1
  Clock1/1 -> Second-->Hour/1
  Second-->Hour/1 -> Add/1

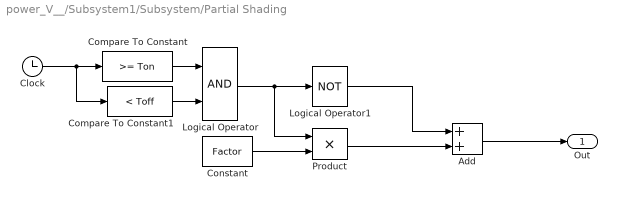
== system power_V__/Subsystem1/Subsystem/Partial Shading ==
  Add : Sum
  Clock : Clock
  Compare To Constant : simulink/Logic and Bit Operations/Compare To Constant  relop=>=  const=Ton  OutDataTypeStr=boolean
  Compare To Constant1 : simulink/Logic and Bit Operations/Compare To Constant  relop=<  const=Toff  OutDataTypeStr=boolean
  Constant : Constant  Value=Factor
  Logical Operator : Logic  AllPortsSameDT=off  OutDataTypeStr=float('double')
  Logical Operator1 : Logic  Operator=NOT  AllPortsSameDT=off  OutDataTypeStr=float('double')
  Product : Product
  Out : Outport  VectorParamsAs1DForOutWhenUnconnected=off
  wires:
  Add/1 -> Out/1
  Product/1 -> Add/2
  Constant/1 -> Product/2
  Compare To Constant/1 -> Logical Operator/1
  Clock/1 -> Compare To Constant1/1, Compare To Constant/1
  Compare To Constant1/1 -> Logical Operator/2
  Logical Operator/1 -> Logical Operator1/1, Product/1
  Logical Operator1/1 -> Add/1

== system power_V__/Subsystem2/Subsystem/Wind profile ==
  1-D Lookup Table : Lookup_n-D  NumberOfTableDimensions=1  BreakpointsForDimension1=V2G.WINDTURBINE.time  BeginIndexSearchUsingPreviousIndexResult=on  Table=V2G.WINDTURBINE.wind  ExtrapMethod=Clip  UseLastTableValue=on  InternalRulePriority=Speed  RndMeth=Simplest  InputSameDT=on
  Add : Sum
  Clock1 : Clock
  Constant1 : Constant
  Second-->Hour : Gain  Gain=1/(60*60)
  " " : Outport  VectorParamsAs1DForOutWhenUnconnected=off
  wires:
  Second-->Hour/1 -> Add/1
  Add/1 -> 1-D Lookup Table/1
  Constant1/1 -> Add/2
  Clock1/1 -> Second-->Hour/1
  1-D Lookup Table/1 -> " "/1

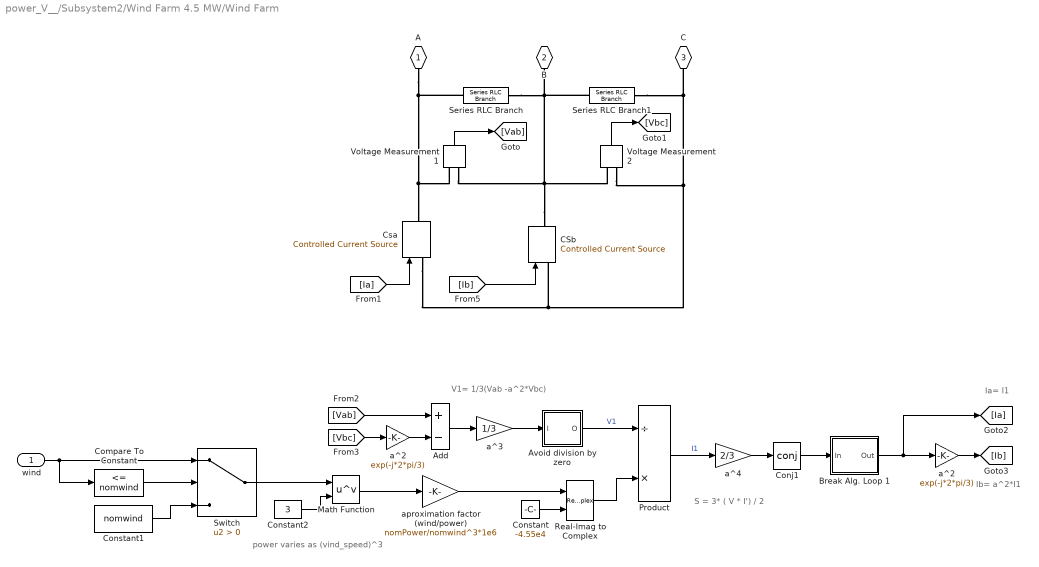
== system power_V__/Subsystem2/Wind Farm 4.5 MW/Wind Farm ==
  note: power varies as (vind_speed)^3
  note: V1= 1/3(Vab -a^2*Vbc)
  note: S = 3* ( V * I') / 2
  note: Ia= I1
  note: Ib= a^2*I1
  "wind " : Inport
  Add : Sum  Inputs=+-
  Avoid division by zero : Subsystem
  Break Alg. Loop 1 : Subsystem
  CSb : powerlib/Electrical Sources/Controlled Current Source  Initialize=on  Source_Type=AC  Amplitude=6286.7  Phase=(-0.5-2*pi/3)*180/pi  Frequency=60  Measurements=Current
      settings: SourceProductName=Simscape Electrical
  Compare To Constant : simulink/Logic and Bit Operations/Compare To Constant  relop=<=  const=nomwind  OutDataTypeStr=boolean
  Conj1 : Math  Operator=conj  SaturateOnIntegerOverflow=on
  Constant : Constant  Value=-4.55e4
  Constant1 : Constant  Value=nomwind
  Constant2 : Constant  Value=3
  Csa : powerlib/Electrical Sources/Controlled Current Source  Initialize=on  Source_Type=AC  Amplitude=6286.7  Phase=-0.5*180/pi  Frequency=60  Measurements=Current
      settings: SourceProductName=Simscape Electrical
  Math Function : Math  Operator=pow  SaturateOnIntegerOverflow=on
  Product : Product  Inputs=/*  SaturateOnIntegerOverflow=on  InputSameDT=on  OutDataTypeStr=Inherit: Same as first input
  Real-Imag to Complex : RealImagToComplex
  Series RLC Branch : powerlib/Elements/Series RLC Branch  LConnTagsString=__new0  RConnTagsString=__new0  BranchType=R  Resistance=1e6  Inductance=1e-3  SetiL0=off  InitialCurrent=0  Capacitance=1e-6  Setx0=off  InitialVoltage=0  Measurements=None
      settings: SourceProductName=Simscape Electrical
  Series RLC Branch1 : powerlib/Elements/Series RLC Branch  LConnTagsString=__new0  RConnTagsString=__new0  BranchType=R  Resistance=1e6  Inductance=1e-3  SetiL0=off  InitialCurrent=0  Capacitance=1e-6  Setx0=off  InitialVoltage=0  Measurements=None
      settings: SourceProductName=Simscape Electrical
  Switch : Switch  Criteria=u2 > Threshold
  Voltage Measurement1 : powerlib/Measurements/Voltage Measurement  PhasorSimulation=on  OutputType=Complex  PSBequivalent=0
      settings: SourceProductName=Simscape Electrical
  Voltage Measurement2 : powerlib/Measurements/Voltage Measurement  PhasorSimulation=on  OutputType=Complex  PSBequivalent=0
      settings: SourceProductName=Simscape Electrical
  a^2 : Gain  Gain=exp(-j*2*pi/3)  SaturateOnIntegerOverflow=on  OutDataTypeStr=Inherit: Same as input  ParamDataTypeStr=Inherit: Same as input
  "a^2 " : Gain  Gain=exp(-j*2*pi/3)  SaturateOnIntegerOverflow=on  OutDataTypeStr=Inherit: Same as input  ParamDataTypeStr=Inherit: Same as input
  a^3 : Gain  Gain=1/3  SaturateOnIntegerOverflow=on  OutDataTypeStr=Inherit: Same as input  ParamDataTypeStr=Inherit: Same as input
  a^4 : Gain  Gain=2/3  SaturateOnIntegerOverflow=on  OutDataTypeStr=Inherit: Same as input  ParamDataTypeStr=Inherit: Same as input
  aproximation factor (wind/power) : Gain  Gain=nomPower/nomwind^3*1e6
  A : PMIOPort  Tag=PMCPort  Side=Right
  B : PMIOPort  Tag=PMCPort  Port=2  Side=Right
  C : PMIOPort  Tag=PMCPort  Port=3  Side=Right
  wires:
  "a^2 "/1 -> Add/2
  [Vbc] -> "a^2 "/1
  Avoid division by zero/1(O) -> Product/1  "V1"
  a^3/1 -> Avoid division by zero/1(I)
  Add/1 -> a^3/1
  [Vab] -> Add/1
  aproximation factor (wind/power)/1 -> Real-Imag to Complex/1
  Constant1/1 -> Switch/3
  Compare To Constant/1 -> Switch/2
  "wind "/1 -> Switch/1, Compare To Constant/1
  Constant/1 -> Real-Imag to Complex/2
  Voltage Measurement1/1 -> [Vab]
  Voltage Measurement2/1 -> [Vbc]
  Real-Imag to Complex/1 -> Product/2
  Product/1 -> a^4/1  "I1"
  a^2/1 -> [Ib]
  Conj1/1 -> Break Alg. Loop 1/1(In)
  a^4/1 -> Conj1/1
  Break Alg. Loop 1/1(Out) -> [Ia], a^2/1
  [Ib] -> CSb/1
  [Ia] -> Csa/1
  Math Function/1 -> aproximation factor (wind/power)/1
  Switch/1 -> Math Function/1
  Constant2/1 -> Math Function/2
  connections:
  A/RConn1 -- Csa/RConn1 -- Voltage Measurement1/LConn1 -- Series RLC Branch/LConn1
  Voltage Measurement2/LConn2 -- Series RLC Branch1/RConn1 -- C/RConn1 -- CSb/LConn1 -- Csa/LConn1
  CSb/RConn1 -- Series RLC Branch/RConn1 -- B/RConn1 -- Series RLC Branch1/LConn1 -- Voltage Measurement2/LConn1 -- Voltage Measurement1/LConn2

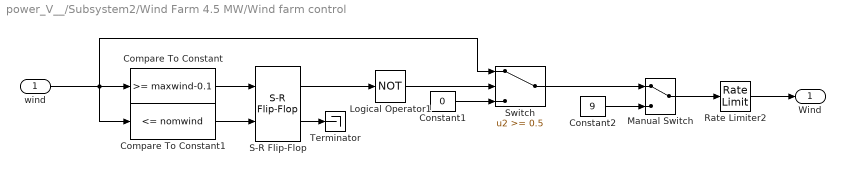
== system power_V__/Subsystem2/Wind Farm 4.5 MW/Wind farm control ==
  "wind " : Inport
  Compare To Constant : simulink/Logic and Bit Operations/Compare To Constant  relop=>=  const=maxwind-0.1  OutDataTypeStr=boolean  ZeroCross=off
  Compare To Constant1 : simulink/Logic and Bit Operations/Compare To Constant  relop=<=  const=nomwind  OutDataTypeStr=boolean  ZeroCross=off
  Constant1 : Constant  Value=0
  Constant2 : Constant  Value=9
  Logical Operator1 : Logic  Operator=NOT  AllPortsSameDT=off  OutDataTypeStr=boolean
  Manual Switch : ManualSwitch
  Rate Limiter2 : RateLimiter  RisingSlewLimit=1e4  FallingSlewLimit=-1e4  SampleTimeMode=inherited
  S-R Flip-Flop : simulink_extras/Flip Flops/S-R Flip-Flop  initial_condition=0
  Switch : Switch  Threshold=0.5  ZeroCross=off
  Terminator : Terminator
  Wind : Outport  VectorParamsAs1DForOutWhenUnconnected=off
  wires:
  "wind "/1 -> Switch/1, Compare To Constant/1, Compare To Constant1/1
  Constant1/1 -> Switch/3
  Logical Operator1/1 -> Switch/2
  S-R Flip-Flop/1 -> Logical Operator1/1
  Compare To Constant1/1 -> S-R Flip-Flop/2
  Compare To Constant/1 -> S-R Flip-Flop/1
  S-R Flip-Flop/2 -> Terminator/1
  Switch/1 -> Manual Switch/1
  Manual Switch/1 -> Rate Limiter2/1
  Constant2/1 -> Manual Switch/2
  Rate Limiter2/1 -> Wind/1

== system power_V__/Load Residential = 10 MW, PF=0.15 ASM = 0.16 MVA /Residential Load/Break Alg. Loop 1/imag ==
  In1 : Inport
  State Space : StateSpace  A=A  B=B  C=C  D=Dd  InitialCondition=X0
  Out1 : Outport  InitialOutput=0  VectorParamsAs1DForOutWhenUnconnected=off
  wires:
  State Space/1 -> Out1/1
  In1/1 -> State Space/1

== system power_V__/Load Residential = 10 MW, PF=0.15 ASM = 0.16 MVA /Residential Load/Break Alg. Loop 1/real ==
  In1 : Inport
  State Space : StateSpace  A=A  B=B  C=C  D=Dd  InitialCondition=X0
  Out1 : Outport  InitialOutput=0  VectorParamsAs1DForOutWhenUnconnected=off
  wires:
  State Space/1 -> Out1/1
  In1/1 -> State Space/1

== system power_V__/Subsystem1/PV Farm 8 MW/PV Farm/Avoid division by zero ==
  I : Inport
  Complex to Magnitude-Angle : ComplexToMagnitudeAngle
  Magnitude-Angle to Complex : MagnitudeAngleToComplex
  Saturation1 : Saturate  UpperLimit=inf  LowerLimit=1e-6
  O : Outport  VectorParamsAs1DForOutWhenUnconnected=off
  wires:
  Complex to Magnitude-Angle/2 -> Magnitude-Angle to Complex/2
  Magnitude-Angle to Complex/1 -> O/1
  Complex to Magnitude-Angle/1 -> Saturation1/1
  Saturation1/1 -> Magnitude-Angle to Complex/1
  I/1 -> Complex to Magnitude-Angle/1
